simulink model "Q5"  (R2022a)
settings: Solver=VariableStepAuto  StartTime=0.0  StopTime=10  RelTol=1e-3
settings Model: Creator=Mahdi Saberi  LastModifiedBy=fatae
settings SolverCC: AlgebraicLoopSolver=TrustRegion
settings DebuggingCC: UnconnectedInputMsg=warning  UnconnectedOutputMsg=warning  UnconnectedLineMsg=warning  SFMachineParentedDataDiag=warning
settings SFSimCC: CustomCodeUndefinedFunction=UseInterfaceOnly

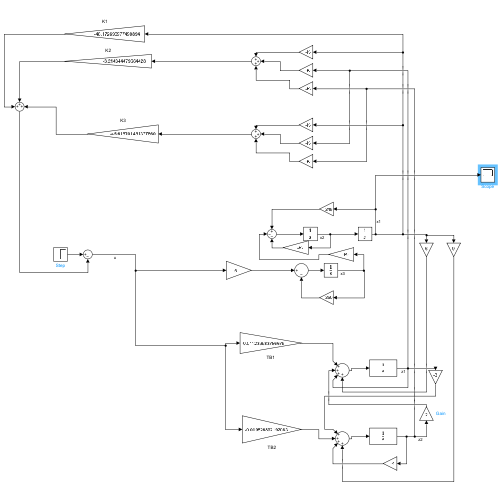
[thumbnail: Simulink's stored preview of the top-level diagram]
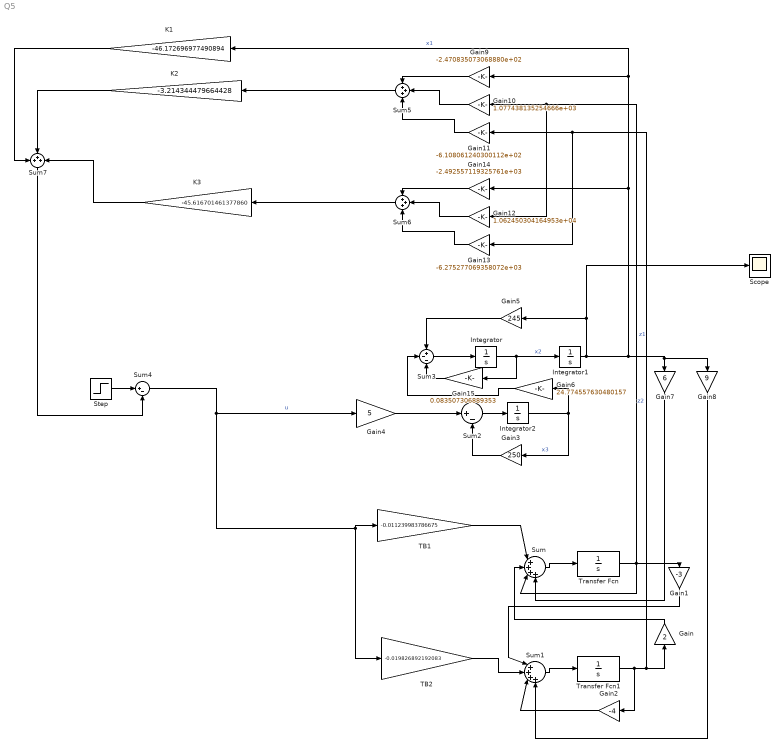
== system Q5 ==
  Gain : Gain  Gain=2
  Gain1 : Gain  Gain=-3
  Gain10 : Gain  Gain=1.077438135254666e+03
  Gain11 : Gain  Gain=-6.108061240300112e+02
  Gain12 : Gain  Gain=1.062450304164953e+04
  Gain13 : Gain  Gain=-6.275277069358072e+03
  Gain14 : Gain  Gain=-2.492557119325761e+03
  Gain15 : Gain  Gain=0.083507306889353
  Gain2 : Gain  Gain=-4
  Gain3 : Gain  Gain=250
  Gain4 : Gain  Gain=5
  Gain5 : Gain  Gain=245
  Gain6 : Gain  Gain=24.774557630480157
  Gain7 : Gain  Gain=6
  Gain8 : Gain  Gain=9
  Gain9 : Gain  Gain=-2.470835073068880e+02
  Integrator : Integrator
  Integrator1 : Integrator
  Integrator2 : Integrator
  K1 : Gain  Gain=-46.172696977490894
  K2 : Gain  Gain=-3.214344479664428
  K3 : Gain  Gain=-45.616701461377860
  Scope : Scope
  Step : Step  Time=0  SampleTime=0
  Sum : Sum  Inputs=|++++
  Sum1 : Sum  Inputs=|++++
  Sum2 : Sum  Inputs=|+-
  Sum3 : Sum  Inputs=+--
  Sum4 : Sum  Inputs=|+-
  Sum5 : Sum  Inputs=3
  Sum6 : Sum  Inputs=3
  Sum7 : Sum  Inputs=3
  TB1 : Gain  Gain=-0.011239983786675
  TB2 : Gain  Gain=-0.019826892192083
  Transfer Fcn : TransferFcn  Denominator=[1 0]
  Transfer Fcn1 : TransferFcn  Denominator=[1 0]
  wires:
  Transfer Fcn/1 -> Gain12/1, Gain10/1, Gain1/1, Sum/3  "z1"
  Transfer Fcn1/1 -> Gain2/1, Gain13/1, Gain11/1, Gain/1  "z2"
  Gain/1 -> Sum/2
  Sum1/1 -> Transfer Fcn1/1
  Gain1/1 -> Sum1/1
  TB1/1 -> Sum/1
  Gain2/1 -> Sum1/3
  TB2/1 -> Sum1/2
  Sum/1 -> Transfer Fcn/1
  Gain6/1 -> Sum3/2
  Sum3/1 -> Integrator/1
  Gain5/1 -> Sum3/1
  Integrator1/1 -> Gain14/1, Gain9/1, K1/1, Gain8/1, Gain7/1, Scope/1, Gain5/1  "x1"
  Sum2/1 -> Integrator2/1
  Gain4/1 -> Sum2/1
  Gain3/1 -> Sum2/2
  Integrator2/1 -> Gain3/1, Gain6/1  "x3"
  Integrator/1 -> Gain15/1, Integrator1/1  "x2"
  Gain7/1 -> Sum/4
  Gain8/1 -> Sum1/4
  Step/1 -> Sum4/1
  Sum4/1 -> Gain4/1, TB2/1, TB1/1  "u"
  Gain9/1 -> Sum5/1
  Gain10/1 -> Sum5/2
  Gain11/1 -> Sum5/3
  Sum5/1 -> K2/1
  Sum6/1 -> K3/1
  Gain13/1 -> Sum6/3
  Gain12/1 -> Sum6/2
  Gain14/1 -> Sum6/1
  K3/1 -> Sum7/3
  K2/1 -> Sum7/2
  K1/1 -> Sum7/1
  Sum7/1 -> Sum4/2
  Gain15/1 -> Sum3/3
